simulink model "DHM"  (R2022a)
settings: Solver=FixedStepDiscrete  StartTime=0.0  StopTime=10.0  FixedStep=0.01  RelTol=1e-3
libraries: simulink x8, DoorHndReq x4, DoorHndDriver x2
settings Model: DataDictionary=DHM.sldd  Creator=liyun  LastModifiedBy=liyun
settings DataIOCC: SaveFormat=StructureWithTime
settings OptimizationCC: DefaultParameterBehavior=Inlined  EnhancedBackFolding=on  PassReuseOutputArgsAs=Individual arguments  ZeroExternalMemoryAtStartup=off  ZeroInternalMemoryAtStartup=off  OptimizeBlockOrder=speed  DifferentSizesBufferReuse=on  OptimizationCustomize=off  EfficientTunableParamExpr=on
settings DebuggingCC: ParameterTunabilityLossMsg=error
settings ModelReferenceCC: ModelReferenceNumInstancesAllowed=Single
settings SFSimCC: MATLABDynamicMemAlloc=off
settings RTWCC: Description=AUTOSAR  SystemTargetFile=autosar.tlc  GenCodeOnly=on  TemplateMakefile=ert_default_tmf
settings CodeAppCC: ForceParamTrailComments=on  IgnoreCustomStorageClasses=off  OperatorAnnotations=on  SimulinkDataObjDesc=on  SFDataObjDesc=on  InsertBlockDesc=on
settings STFCustomTargetCC: TargetLangStandard=C99 (ISO)  MultiwordLength=256  ParMdlRefBuildCompliant=on  CompOptLevelCompliant=on  IncludeMdlTerminateFcn=off  CombineOutputUpdateFcns=on  SuppressErrorStatus=on  ERTCustomFileBanners=on  SupportNonFinite=off  SupportComplex=off  SupportContinuousTime=off  SupportNonInlinedSFcns=off  RemoveResetFunc=on  MATLABClassNameForMDSCustomization=Simulink.SoftwareTarget.ERTCustomization  AutosarCompliant=on  GRTInterface=off  UseToolchainInfoCompliant=on  LookupTableObjectStructAxisOrder=2,1,3,4,...  LUTObjectStructOrderEvenSpacing=Size,Table,Breakpoints  SystemTargetFile=autosar.tlc
settings ERTTargetCC: TargetLangStandard=C99 (ISO)  ConcurrentExecutionCompliant=off  IncludeMdlTerminateFcn=off  SuppressErrorStatus=on  SupportNonFinite=off  SupportComplex=off  ModelStepFunctionPrototypeControlCompliant=off  CPPClassGenCompliant=off  AutosarCompliant=on  LookupTableObjectStructAxisOrder=2,1,3,4,...  LUTObjectStructOrderEvenSpacing=Size,Table,Breakpoints  InlinedParameterPlacement=NonHierarchical  ERTCustomFileTemplate=example_file_process.tlc

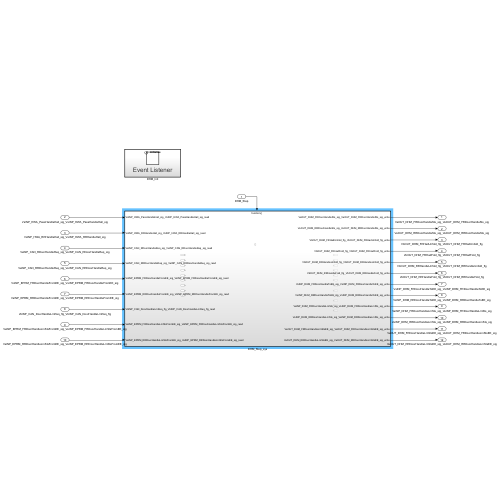
[thumbnail: Simulink's stored preview of the top-level diagram]
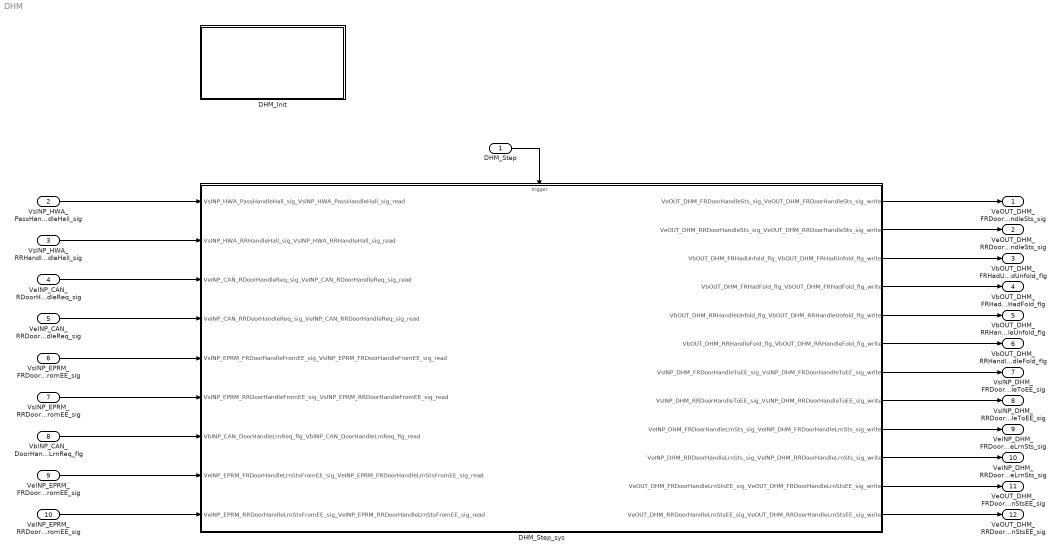
== system DHM ==
  DHM_Step : Inport  SampleTime=0.01  OutputFunctionCall=on
  VsINP_HWA_PassHandleHall_sig_VsINP_HWA_PassHandleHall_sig : Inport  Port=2  OutDataTypeStr=SInt16  PortDimensions=1
  VsINP_HWA_RRHandleHall_sig_VsINP_HWA_RRHandleHall_sig : Inport  Port=3  OutDataTypeStr=SInt16  PortDimensions=1
  VeINP_CAN_RDoorHandleReq_sig_VeINP_CAN_RDoorHandleReq_sig : Inport  Port=4  OutDataTypeStr=UInt8  PortDimensions=1
  VeINP_CAN_RRDoorHandleReq_sig_VeINP_CAN_RRDoorHandleReq_sig : Inport  Port=5  OutDataTypeStr=UInt8  PortDimensions=1
  VsINP_EPRM_FRDoorHandleFromEE_sig_VsINP_EPRM_FRDoorHandleFromEE_sig : Inport  Port=6  OutDataTypeStr=SInt16  PortDimensions=1
  VsINP_EPRM_RRDoorHandleFromEE_sig_VsINP_EPRM_RRDoorHandleFromEE_sig : Inport  Port=7  OutDataTypeStr=SInt16  PortDimensions=1
  VbINP_CAN_DoorHandleLrnReq_flg_VbINP_CAN_DoorHandleLrnReq_flg : Inport  Port=8  OutDataTypeStr=Boolean  PortDimensions=1
  VeINP_EPRM_FRDoorHandleLrnStsFromEE_sig_VeINP_EPRM_FRDoorHandleLrnStsFromEE_sig : Inport  Port=9  OutDataTypeStr=UInt8  PortDimensions=1
  VeINP_EPRM_RRDoorHandleLrnStsFromEE_sig_VeINP_EPRM_RRDoorHandleLrnStsFromEE_sig : Inport  Port=10  OutDataTypeStr=UInt8  PortDimensions=1
  DHM_Init : Subsystem
  DHM_Step_sys : Subsystem
  VeOUT_DHM_FRDoorHandleSts_sig_VeOUT_DHM_FRDoorHandleSts_sig : Outport  OutDataTypeStr=UInt8  PortDimensions=1
  VeOUT_DHM_RRDoorHandleSts_sig_VeOUT_DHM_RRDoorHandleSts_sig : Outport  Port=2  OutDataTypeStr=UInt8  PortDimensions=1
  VbOUT_DHM_FRHadUnfold_flg_VbOUT_DHM_FRHadUnfold_flg : Outport  Port=3  OutDataTypeStr=Boolean  PortDimensions=1
  VbOUT_DHM_FRHadFold_flg_VbOUT_DHM_FRHadFold_flg : Outport  Port=4  OutDataTypeStr=Boolean  PortDimensions=1
  VbOUT_DHM_RRHandleUnfold_flg_VbOUT_DHM_RRHandleUnfold_flg : Outport  Port=5  OutDataTypeStr=Boolean  PortDimensions=1
  VbOUT_DHM_RRHandleFold_flg_VbOUT_DHM_RRHandleFold_flg : Outport  Port=6  OutDataTypeStr=Boolean  PortDimensions=1
  VsINP_DHM_FRDoorHandleToEE_sig_VsINP_DHM_FRDoorHandleToEE_sig : Outport  Port=7  OutDataTypeStr=SInt16  PortDimensions=1
  VsINP_DHM_RRDoorHandleToEE_sig_VsINP_DHM_RRDoorHandleToEE_sig : Outport  Port=8  OutDataTypeStr=SInt16  PortDimensions=1
  VeINP_DHM_FRDoorHandleLrnSts_sig_VeINP_DHM_FRDoorHandleLrnSts_sig : Outport  Port=9  OutDataTypeStr=UInt8  PortDimensions=1
  VeINP_DHM_RRDoorHandleLrnSts_sig_VeINP_DHM_RRDoorHandleLrnSts_sig : Outport  Port=10  OutDataTypeStr=UInt8  PortDimensions=1
  VeOUT_DHM_FRDoorHandleLrnStsEE_sig_VeOUT_DHM_FRDoorHandleLrnStsEE_sig : Outport  Port=11  OutDataTypeStr=UInt8  PortDimensions=1
  VeOUT_DHM_RRDoorHandleLrnStsEE_sig_VeOUT_DHM_RRDoorHandleLrnStsEE_sig : Outport  Port=12  OutDataTypeStr=UInt8  PortDimensions=1
  wires:
  VsINP_HWA_PassHandleHall_sig_VsINP_HWA_PassHandleHall_sig/1 -> DHM_Step_sys/1(VsINP_HWA_PassHandleHall_sig_VsINP_HWA_PassHandleHall_sig_read)
  VsINP_HWA_RRHandleHall_sig_VsINP_HWA_RRHandleHall_sig/1 -> DHM_Step_sys/2(VsINP_HWA_RRHandleHall_sig_VsINP_HWA_RRHandleHall_sig_read)
  VeINP_CAN_RDoorHandleReq_sig_VeINP_CAN_RDoorHandleReq_sig/1 -> DHM_Step_sys/3(VeINP_CAN_RDoorHandleReq_sig_VeINP_CAN_RDoorHandleReq_sig_read)
  VeINP_CAN_RRDoorHandleReq_sig_VeINP_CAN_RRDoorHandleReq_sig/1 -> DHM_Step_sys/4(VeINP_CAN_RRDoorHandleReq_sig_VeINP_CAN_RRDoorHandleReq_sig_read)
  VsINP_EPRM_FRDoorHandleFromEE_sig_VsINP_EPRM_FRDoorHandleFromEE_sig/1 -> DHM_Step_sys/5(VsINP_EPRM_FRDoorHandleFromEE_sig_VsINP_EPRM_FRDoorHandleFromEE_sig_read)
  VsINP_EPRM_RRDoorHandleFromEE_sig_VsINP_EPRM_RRDoorHandleFromEE_sig/1 -> DHM_Step_sys/6(VsINP_EPRM_RRDoorHandleFromEE_sig_VsINP_EPRM_RRDoorHandleFromEE_sig_read)
  VbINP_CAN_DoorHandleLrnReq_flg_VbINP_CAN_DoorHandleLrnReq_flg/1 -> DHM_Step_sys/7(VbINP_CAN_DoorHandleLrnReq_flg_VbINP_CAN_DoorHandleLrnReq_flg_read)
  VeINP_EPRM_FRDoorHandleLrnStsFromEE_sig_VeINP_EPRM_FRDoorHandleLrnStsFromEE_sig/1 -> DHM_Step_sys/8(VeINP_EPRM_FRDoorHandleLrnStsFromEE_sig_VeINP_EPRM_FRDoorHandleLrnStsFromEE_sig_read)
  VeINP_EPRM_RRDoorHandleLrnStsFromEE_sig_VeINP_EPRM_RRDoorHandleLrnStsFromEE_sig/1 -> DHM_Step_sys/9(VeINP_EPRM_RRDoorHandleLrnStsFromEE_sig_VeINP_EPRM_RRDoorHandleLrnStsFromEE_sig_read)
  DHM_Step_sys/1(VeOUT_DHM_FRDoorHandleSts_sig_VeOUT_DHM_FRDoorHandleSts_sig_write) -> VeOUT_DHM_FRDoorHandleSts_sig_VeOUT_DHM_FRDoorHandleSts_sig/1
  DHM_Step_sys/2(VeOUT_DHM_RRDoorHandleSts_sig_VeOUT_DHM_RRDoorHandleSts_sig_write) -> VeOUT_DHM_RRDoorHandleSts_sig_VeOUT_DHM_RRDoorHandleSts_sig/1
  DHM_Step_sys/3(VbOUT_DHM_FRHadUnfold_flg_VbOUT_DHM_FRHadUnfold_flg_write) -> VbOUT_DHM_FRHadUnfold_flg_VbOUT_DHM_FRHadUnfold_flg/1
  DHM_Step_sys/4(VbOUT_DHM_FRHadFold_flg_VbOUT_DHM_FRHadFold_flg_write) -> VbOUT_DHM_FRHadFold_flg_VbOUT_DHM_FRHadFold_flg/1
  DHM_Step_sys/5(VbOUT_DHM_RRHandleUnfold_flg_VbOUT_DHM_RRHandleUnfold_flg_write) -> VbOUT_DHM_RRHandleUnfold_flg_VbOUT_DHM_RRHandleUnfold_flg/1
  DHM_Step_sys/6(VbOUT_DHM_RRHandleFold_flg_VbOUT_DHM_RRHandleFold_flg_write) -> VbOUT_DHM_RRHandleFold_flg_VbOUT_DHM_RRHandleFold_flg/1
  DHM_Step_sys/7(VsINP_DHM_FRDoorHandleToEE_sig_VsINP_DHM_FRDoorHandleToEE_sig_write) -> VsINP_DHM_FRDoorHandleToEE_sig_VsINP_DHM_FRDoorHandleToEE_sig/1
  DHM_Step_sys/8(VsINP_DHM_RRDoorHandleToEE_sig_VsINP_DHM_RRDoorHandleToEE_sig_write) -> VsINP_DHM_RRDoorHandleToEE_sig_VsINP_DHM_RRDoorHandleToEE_sig/1
  DHM_Step_sys/9(VeINP_DHM_FRDoorHandleLrnSts_sig_VeINP_DHM_FRDoorHandleLrnSts_sig_write) -> VeINP_DHM_FRDoorHandleLrnSts_sig_VeINP_DHM_FRDoorHandleLrnSts_sig/1
  DHM_Step_sys/10(VeINP_DHM_RRDoorHandleLrnSts_sig_VeINP_DHM_RRDoorHandleLrnSts_sig_write) -> VeINP_DHM_RRDoorHandleLrnSts_sig_VeINP_DHM_RRDoorHandleLrnSts_sig/1
  DHM_Step_sys/11(VeOUT_DHM_FRDoorHandleLrnStsEE_sig_VeOUT_DHM_FRDoorHandleLrnStsEE_sig_write) -> VeOUT_DHM_FRDoorHandleLrnStsEE_sig_VeOUT_DHM_FRDoorHandleLrnStsEE_sig/1
  DHM_Step_sys/12(VeOUT_DHM_RRDoorHandleLrnStsEE_sig_VeOUT_DHM_RRDoorHandleLrnStsEE_sig_write) -> VeOUT_DHM_RRDoorHandleLrnStsEE_sig_VeOUT_DHM_RRDoorHandleLrnStsEE_sig/1
  DHM_Step/1 -> DHM_Step_sys/Trigger

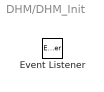
== system DHM/DHM_Init ==
  Event Listener : EventListener  EventName=reset

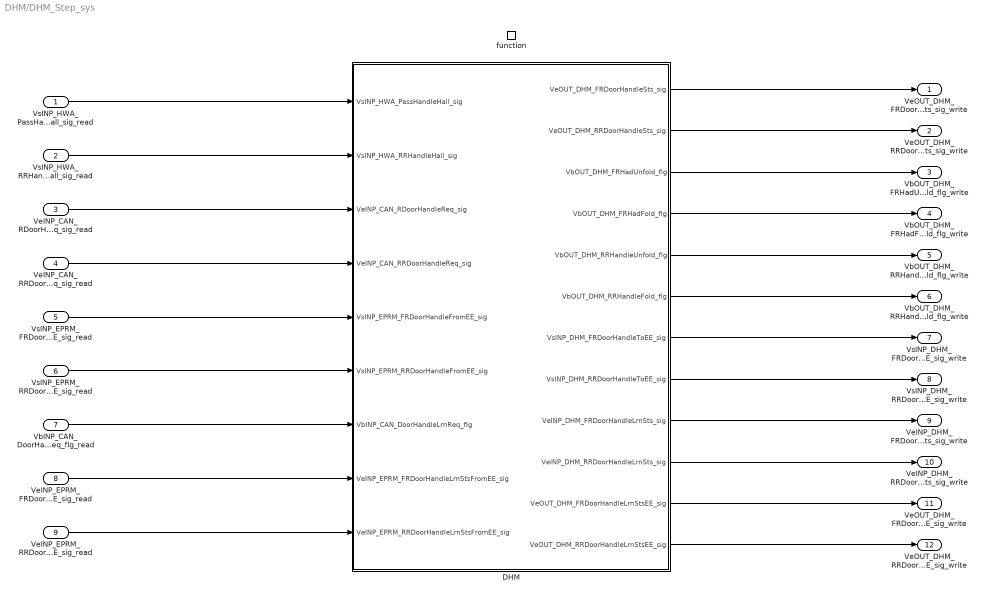
== system DHM/DHM_Step_sys ==
  VsINP_HWA_PassHandleHall_sig_VsINP_HWA_PassHandleHall_sig_read : Inport
  VsINP_HWA_RRHandleHall_sig_VsINP_HWA_RRHandleHall_sig_read : Inport  Port=2
  VeINP_CAN_RDoorHandleReq_sig_VeINP_CAN_RDoorHandleReq_sig_read : Inport  Port=3
  VeINP_CAN_RRDoorHandleReq_sig_VeINP_CAN_RRDoorHandleReq_sig_read : Inport  Port=4
  VsINP_EPRM_FRDoorHandleFromEE_sig_VsINP_EPRM_FRDoorHandleFromEE_sig_read : Inport  Port=5
  VsINP_EPRM_RRDoorHandleFromEE_sig_VsINP_EPRM_RRDoorHandleFromEE_sig_read : Inport  Port=6
  VbINP_CAN_DoorHandleLrnReq_flg_VbINP_CAN_DoorHandleLrnReq_flg_read : Inport  Port=7
  VeINP_EPRM_FRDoorHandleLrnStsFromEE_sig_VeINP_EPRM_FRDoorHandleLrnStsFromEE_sig_read : Inport  Port=8
  VeINP_EPRM_RRDoorHandleLrnStsFromEE_sig_VeINP_EPRM_RRDoorHandleLrnStsFromEE_sig_read : Inport  Port=9
  function : TriggerPort  TriggerType=function-call  VariantControl=(inherit)  SampleTimeType=periodic  SampleTime=-1
  DHM : Subsystem
  VeOUT_DHM_FRDoorHandleSts_sig_VeOUT_DHM_FRDoorHandleSts_sig_write : Outport
      settings: EnsureOutportIsVirtual=on
  VeOUT_DHM_RRDoorHandleSts_sig_VeOUT_DHM_RRDoorHandleSts_sig_write : Outport  Port=2
      settings: EnsureOutportIsVirtual=on
  VbOUT_DHM_FRHadUnfold_flg_VbOUT_DHM_FRHadUnfold_flg_write : Outport  Port=3
      settings: EnsureOutportIsVirtual=on
  VbOUT_DHM_FRHadFold_flg_VbOUT_DHM_FRHadFold_flg_write : Outport  Port=4
      settings: EnsureOutportIsVirtual=on
  VbOUT_DHM_RRHandleUnfold_flg_VbOUT_DHM_RRHandleUnfold_flg_write : Outport  Port=5
      settings: EnsureOutportIsVirtual=on
  VbOUT_DHM_RRHandleFold_flg_VbOUT_DHM_RRHandleFold_flg_write : Outport  Port=6
      settings: EnsureOutportIsVirtual=on
  VsINP_DHM_FRDoorHandleToEE_sig_VsINP_DHM_FRDoorHandleToEE_sig_write : Outport  Port=7
      settings: EnsureOutportIsVirtual=on
  VsINP_DHM_RRDoorHandleToEE_sig_VsINP_DHM_RRDoorHandleToEE_sig_write : Outport  Port=8
      settings: EnsureOutportIsVirtual=on
  VeINP_DHM_FRDoorHandleLrnSts_sig_VeINP_DHM_FRDoorHandleLrnSts_sig_write : Outport  Port=9
      settings: EnsureOutportIsVirtual=on
  VeINP_DHM_RRDoorHandleLrnSts_sig_VeINP_DHM_RRDoorHandleLrnSts_sig_write : Outport  Port=10
      settings: EnsureOutportIsVirtual=on
  VeOUT_DHM_FRDoorHandleLrnStsEE_sig_VeOUT_DHM_FRDoorHandleLrnStsEE_sig_write : Outport  Port=11
      settings: EnsureOutportIsVirtual=on
  VeOUT_DHM_RRDoorHandleLrnStsEE_sig_VeOUT_DHM_RRDoorHandleLrnStsEE_sig_write : Outport  Port=12
      settings: EnsureOutportIsVirtual=on
  wires:
  VsINP_HWA_PassHandleHall_sig_VsINP_HWA_PassHandleHall_sig_read/1 -> DHM/1(VsINP_HWA_PassHandleHall_sig)
  VsINP_HWA_RRHandleHall_sig_VsINP_HWA_RRHandleHall_sig_read/1 -> DHM/2(VsINP_HWA_RRHandleHall_sig)
  VeINP_CAN_RDoorHandleReq_sig_VeINP_CAN_RDoorHandleReq_sig_read/1 -> DHM/3(VeINP_CAN_RDoorHandleReq_sig)
  VeINP_CAN_RRDoorHandleReq_sig_VeINP_CAN_RRDoorHandleReq_sig_read/1 -> DHM/4(VeINP_CAN_RRDoorHandleReq_sig)
  VsINP_EPRM_FRDoorHandleFromEE_sig_VsINP_EPRM_FRDoorHandleFromEE_sig_read/1 -> DHM/5(VsINP_EPRM_FRDoorHandleFromEE_sig)
  VsINP_EPRM_RRDoorHandleFromEE_sig_VsINP_EPRM_RRDoorHandleFromEE_sig_read/1 -> DHM/6(VsINP_EPRM_RRDoorHandleFromEE_sig)
  VbINP_CAN_DoorHandleLrnReq_flg_VbINP_CAN_DoorHandleLrnReq_flg_read/1 -> DHM/7(VbINP_CAN_DoorHandleLrnReq_flg)
  VeINP_EPRM_FRDoorHandleLrnStsFromEE_sig_VeINP_EPRM_FRDoorHandleLrnStsFromEE_sig_read/1 -> DHM/8(VeINP_EPRM_FRDoorHandleLrnStsFromEE_sig)
  VeINP_EPRM_RRDoorHandleLrnStsFromEE_sig_VeINP_EPRM_RRDoorHandleLrnStsFromEE_sig_read/1 -> DHM/9(VeINP_EPRM_RRDoorHandleLrnStsFromEE_sig)
  DHM/2(VeOUT_DHM_RRDoorHandleSts_sig) -> VeOUT_DHM_RRDoorHandleSts_sig_VeOUT_DHM_RRDoorHandleSts_sig_write/1
  DHM/3(VbOUT_DHM_FRHadUnfold_flg) -> VbOUT_DHM_FRHadUnfold_flg_VbOUT_DHM_FRHadUnfold_flg_write/1
  DHM/1(VeOUT_DHM_FRDoorHandleSts_sig) -> VeOUT_DHM_FRDoorHandleSts_sig_VeOUT_DHM_FRDoorHandleSts_sig_write/1
  DHM/4(VbOUT_DHM_FRHadFold_flg) -> VbOUT_DHM_FRHadFold_flg_VbOUT_DHM_FRHadFold_flg_write/1
  DHM/5(VbOUT_DHM_RRHandleUnfold_flg) -> VbOUT_DHM_RRHandleUnfold_flg_VbOUT_DHM_RRHandleUnfold_flg_write/1
  DHM/6(VbOUT_DHM_RRHandleFold_flg) -> VbOUT_DHM_RRHandleFold_flg_VbOUT_DHM_RRHandleFold_flg_write/1
  DHM/7(VsINP_DHM_FRDoorHandleToEE_sig) -> VsINP_DHM_FRDoorHandleToEE_sig_VsINP_DHM_FRDoorHandleToEE_sig_write/1
  DHM/8(VsINP_DHM_RRDoorHandleToEE_sig) -> VsINP_DHM_RRDoorHandleToEE_sig_VsINP_DHM_RRDoorHandleToEE_sig_write/1
  DHM/9(VeINP_DHM_FRDoorHandleLrnSts_sig) -> VeINP_DHM_FRDoorHandleLrnSts_sig_VeINP_DHM_FRDoorHandleLrnSts_sig_write/1
  DHM/10(VeINP_DHM_RRDoorHandleLrnSts_sig) -> VeINP_DHM_RRDoorHandleLrnSts_sig_VeINP_DHM_RRDoorHandleLrnSts_sig_write/1
  DHM/11(VeOUT_DHM_FRDoorHandleLrnStsEE_sig) -> VeOUT_DHM_FRDoorHandleLrnStsEE_sig_VeOUT_DHM_FRDoorHandleLrnStsEE_sig_write/1
  DHM/12(VeOUT_DHM_RRDoorHandleLrnStsEE_sig) -> VeOUT_DHM_RRDoorHandleLrnStsEE_sig_VeOUT_DHM_RRDoorHandleLrnStsEE_sig_write/1

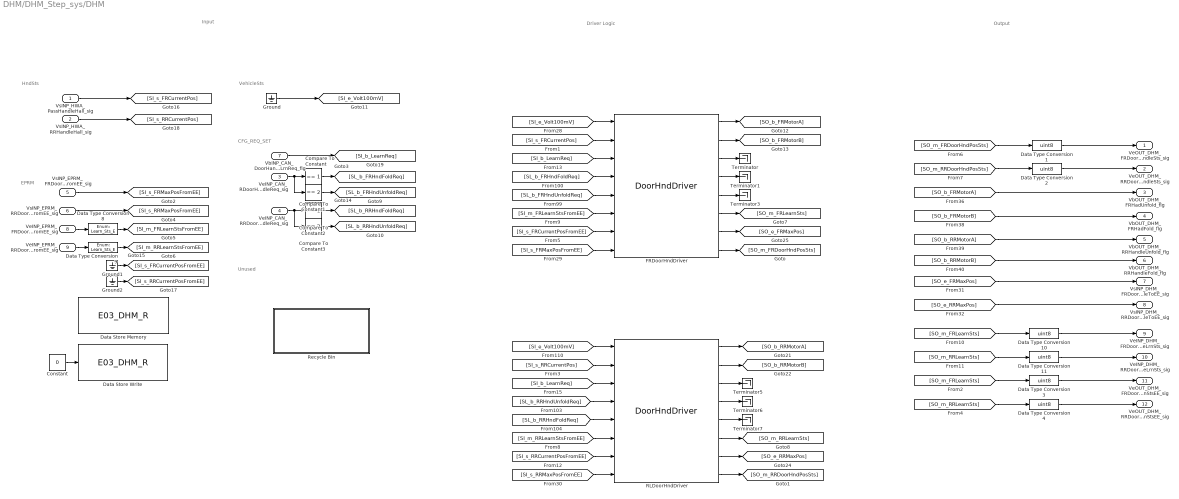
== system DHM/DHM_Step_sys/DHM ==
  note: HndSts
  note: Output
  note: Driver Logic
  note: Input
  note: VehicleSts
  note: Unused
  note: CFG_REQ_SET
  note: EPRM
  VsINP_HWA_PassHandleHall_sig : Inport
  VsINP_HWA_RRHandleHall_sig : Inport  Port=2
  VeINP_CAN_RDoorHandleReq_sig : Inport  Port=3
  VeINP_CAN_RRDoorHandleReq_sig : Inport  Port=4
  VsINP_EPRM_FRDoorHandleFromEE_sig : Inport  Port=5
  VsINP_EPRM_RRDoorHandleFromEE_sig : Inport  Port=6
  VbINP_CAN_DoorHandleLrnReq_flg : Inport  Port=7
  VeINP_EPRM_FRDoorHandleLrnStsFromEE_sig : Inport  Port=8
  VeINP_EPRM_RRDoorHandleLrnStsFromEE_sig : Inport  Port=9
  Compare To Constant : simulink/Logic and Bit Operations/Compare To Constant  relop===  const=1  OutDataTypeStr=boolean
  Compare To Constant1 : simulink/Logic and Bit Operations/Compare To Constant  relop===  const=2  OutDataTypeStr=boolean
  Compare To Constant2 : simulink/Logic and Bit Operations/Compare To Constant  relop===  const=1  OutDataTypeStr=boolean
  Compare To Constant3 : simulink/Logic and Bit Operations/Compare To Constant  relop===  const=2  OutDataTypeStr=boolean
  Constant : Constant  Value=0  OutDataTypeStr=uint8
  Data Store Memory : DataStoreMemory  DataStoreName=E03_DHM_R  WriteAfterWriteMsg=warning  ShowAdditionalParam=off  OutDataTypeStr=uint8
  Data Store Write : DataStoreWrite  DataStoreName=E03_DHM_R  IndexOptions=Index vector (dialog)  Indices=1  OutputSizes=1
  Data Type Conversion{1..4,10..11} (6 alike) : DataTypeConversion  OutDataTypeStr=uint8  SaturateOnIntegerOverflow=off  RndMeth=Floor
  Data Type Conversion8 : DataTypeConversion  OutDataTypeStr=Enum: Learn_Sts_E  SaturateOnIntegerOverflow=off  RndMeth=Floor
  Data Type Conversion9 : DataTypeConversion  OutDataTypeStr=Enum: Learn_Sts_E  SaturateOnIntegerOverflow=off  RndMeth=Floor
  FRDoorHndDriver : DoorHndDriver/DoorHndDriver  SystemSampleTime=-1  VariantActivationTime=update diagram  Latency=0  AutoFrameSizeCalculation=off
  Ground : Ground
  Ground1 : Ground
  Ground2 : Ground
  RLDoorHndDriver : DoorHndDriver/DoorHndDriver  SystemSampleTime=-1  VariantActivationTime=update diagram  Latency=0  AutoFrameSizeCalculation=off
  Recycle Bin : Subsystem
  Terminator{,1,3,5..7} (6 alike) : Terminator
  VeOUT_DHM_FRDoorHandleSts_sig : Outport
  VeOUT_DHM_RRDoorHandleSts_sig : Outport  Port=2
  VbOUT_DHM_FRHadUnfold_flg : Outport  Port=3
  VbOUT_DHM_FRHadFold_flg : Outport  Port=4
  VbOUT_DHM_RRHandleUnfold_flg : Outport  Port=5
  VbOUT_DHM_RRHandleFold_flg : Outport  Port=6
  VsINP_DHM_FRDoorHandleToEE_sig : Outport  Port=7
  VsINP_DHM_RRDoorHandleToEE_sig : Outport  Port=8
  VeINP_DHM_FRDoorHandleLrnSts_sig : Outport  Port=9
  VeINP_DHM_RRDoorHandleLrnSts_sig : Outport  Port=10
  VeOUT_DHM_FRDoorHandleLrnStsEE_sig : Outport  Port=11
  VeOUT_DHM_RRDoorHandleLrnStsEE_sig : Outport  Port=12
  wires:
  [SI_e_Volt100mV] -> FRDoorHndDriver/1
  [SI_e_Volt100mV] -> RLDoorHndDriver/1
  Ground/1 -> [SI_e_Volt100mV]
  Constant/1 -> Data Store Write/1
  VsINP_HWA_PassHandleHall_sig/1 -> [SI_s_FRCurrentPos]
  VsINP_HWA_RRHandleHall_sig/1 -> [SI_s_RRCurrentPos]
  [SI_s_FRCurrentPos] -> FRDoorHndDriver/2
  [SI_s_RRCurrentPos] -> RLDoorHndDriver/2
  VbINP_CAN_DoorHandleLrnReq_flg/1 -> [SI_b_LearnReq]
  [SI_b_LearnReq] -> FRDoorHndDriver/3
  [SI_b_LearnReq] -> RLDoorHndDriver/3
  VsINP_EPRM_FRDoorHandleFromEE_sig/1 -> [SI_s_FRMaxPosFromEE]
  VsINP_EPRM_RRDoorHandleFromEE_sig/1 -> [SI_s_RRMaxPosFromEE]
  [SO_e_RRMaxPos] -> VsINP_DHM_RRDoorHandleToEE_sig/1
  [SO_e_FRMaxPos] -> VsINP_DHM_FRDoorHandleToEE_sig/1
  [SO_b_FRMotorA] -> VbOUT_DHM_FRHadUnfold_flg/1
  [SO_b_FRMotorB] -> VbOUT_DHM_FRHadFold_flg/1
  [SO_b_RRMotorA] -> VbOUT_DHM_RRHandleUnfold_flg/1
  [SO_b_RRMotorB] -> VbOUT_DHM_RRHandleFold_flg/1
  FRDoorHndDriver/1 -> [SO_b_FRMotorA]
  FRDoorHndDriver/2 -> [SO_b_FRMotorB]
  [SI_m_FRLearnStsFromEE] -> FRDoorHndDriver/6
  [SL_b_FRHndUnfoldReq] -> FRDoorHndDriver/5
  [SL_b_FRHndFoldReq] -> FRDoorHndDriver/4
  [SI_m_RRLearnStsFromEE] -> RLDoorHndDriver/6
  [SL_b_RRHndFoldReq] -> RLDoorHndDriver/5
  [SL_b_RRHndUnfoldReq] -> RLDoorHndDriver/4
  RLDoorHndDriver/1 -> [SO_b_RRMotorA]
  RLDoorHndDriver/2 -> [SO_b_RRMotorB]
  [SO_m_FRDoorHndPosSts] -> Data Type Conversion1/1
  Data Type Conversion1/1 -> VeOUT_DHM_FRDoorHandleSts_sig/1
  Data Type Conversion2/1 -> VeOUT_DHM_RRDoorHandleSts_sig/1
  [SO_m_RRDoorHndPosSts] -> Data Type Conversion2/1
  VeINP_EPRM_FRDoorHandleLrnStsFromEE_sig/1 -> Data Type Conversion8/1
  Data Type Conversion8/1 -> [SI_m_FRLearnStsFromEE]
  VeINP_EPRM_RRDoorHandleLrnStsFromEE_sig/1 -> Data Type Conversion9/1
  Data Type Conversion9/1 -> [SI_m_RRLearnStsFromEE]
  [SO_m_FRLearnSts] -> Data Type Conversion10/1
  Data Type Conversion10/1 -> VeINP_DHM_FRDoorHandleLrnSts_sig/1
  [SO_m_RRLearnSts] -> Data Type Conversion11/1
  Data Type Conversion11/1 -> VeINP_DHM_RRDoorHandleLrnSts_sig/1
  VeINP_CAN_RDoorHandleReq_sig/1 -> Compare To Constant1/1, Compare To Constant/1
  Compare To Constant/1 -> [SL_b_FRHndFoldReq]
  Compare To Constant1/1 -> [SL_b_FRHndUnfoldReq]
  Compare To Constant3/1 -> [SL_b_RRHndUnfoldReq]
  Compare To Constant2/1 -> [SL_b_RRHndFoldReq]
  VeINP_CAN_RRDoorHandleReq_sig/1 -> Compare To Constant3/1, Compare To Constant2/1
  Data Type Conversion3/1 -> VeOUT_DHM_FRDoorHandleLrnStsEE_sig/1
  [SO_m_RRLearnSts] -> Data Type Conversion4/1
  Data Type Conversion4/1 -> VeOUT_DHM_RRDoorHandleLrnStsEE_sig/1
  [SO_m_FRLearnSts] -> Data Type Conversion3/1
  RLDoorHndDriver/3 -> Terminator5/1
  RLDoorHndDriver/4 -> Terminator6/1
  FRDoorHndDriver/3 -> Terminator/1
  FRDoorHndDriver/4 -> Terminator1/1
  FRDoorHndDriver/7 -> [SO_e_FRMaxPos]
  FRDoorHndDriver/6 -> [SO_m_FRLearnSts]
  FRDoorHndDriver/8 -> [SO_m_FRDoorHndPosSts]
  FRDoorHndDriver/5 -> Terminator3/1
  [SI_s_FRMaxPosFromEE] -> FRDoorHndDriver/8
  [SI_s_FRCurrentPosFromEE] -> FRDoorHndDriver/7
  RLDoorHndDriver/7 -> [SO_e_RRMaxPos]
  RLDoorHndDriver/6 -> [SO_m_RRLearnSts]
  RLDoorHndDriver/8 -> [SO_m_RRDoorHndPosSts]
  RLDoorHndDriver/5 -> Terminator7/1
  [SI_s_RRCurrentPosFromEE] -> RLDoorHndDriver/7
  [SI_s_RRMaxPosFromEE] -> RLDoorHndDriver/8
  Ground2/1 -> [SI_s_RRCurrentPosFromEE]
  Ground1/1 -> [SI_s_FRCurrentPosFromEE]

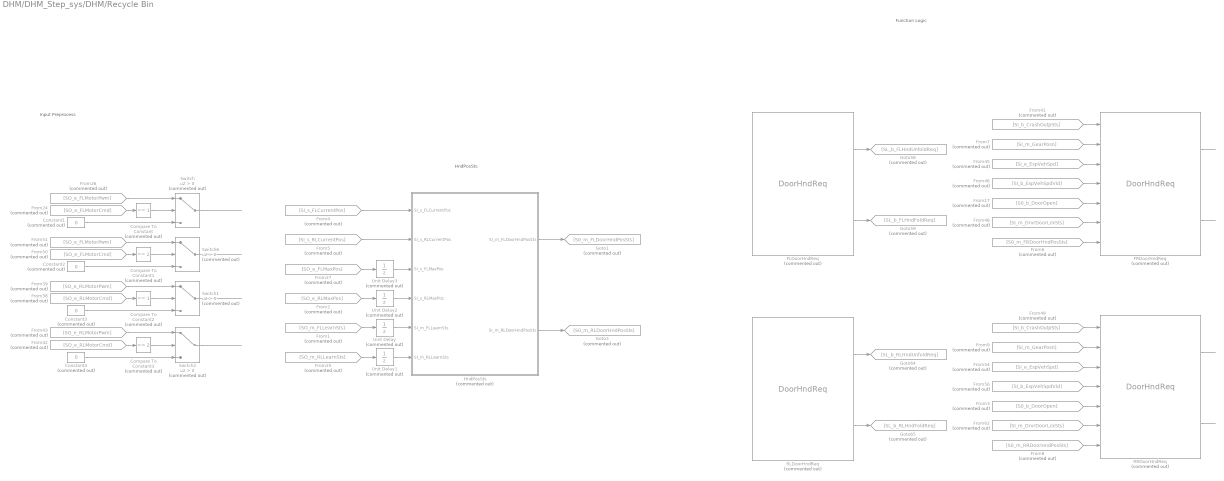
== system DHM/DHM_Step_sys/DHM/Recycle Bin ==
  note: Input Preprocess
  note: HndPosSts
  note: Function Logic
  Compare To Constant : simulink/Logic and Bit Operations/Compare To Constant  Commented=on  relop===  const=1  OutDataTypeStr=boolean
  Compare To Constant1 : simulink/Logic and Bit Operations/Compare To Constant  Commented=on  relop===  const=2  OutDataTypeStr=boolean
  Compare To Constant2 : simulink/Logic and Bit Operations/Compare To Constant  Commented=on  relop===  const=1  OutDataTypeStr=boolean
  Compare To Constant3 : simulink/Logic and Bit Operations/Compare To Constant  Commented=on  relop===  const=2  OutDataTypeStr=boolean
  Constant{1..4} (4 alike) : Constant  Commented=on  Value=0
  FLDoorHndReq : DoorHndReq/DoorHndReq  Commented=on  SystemSampleTime=-1  VariantActivationTime=update diagram  Latency=0  AutoFrameSizeCalculation=off
  FRDoorHndReq : DoorHndReq/DoorHndReq  Commented=on  SystemSampleTime=-1  VariantActivationTime=update diagram  Latency=0  AutoFrameSizeCalculation=off
  From1 : From  Commented=on  GotoTag=SO_m_FLLearnSts
  From17 : From  Commented=on  GotoTag=S0_b_DoorOpen
  From2 : From  Commented=on  GotoTag=SO_e_RLMaxPos
  From24 : From  Commented=on  GotoTag=SO_e_FLMotorCmd
  From25 : From  Commented=on  GotoTag=SO_m_RLLearnSts
  From26 : From  Commented=on  GotoTag=SO_e_FLMotorPwm
  From27 : From  Commented=on  GotoTag=SO_e_FLMaxPos
  From3 : From  Commented=on  GotoTag=S0_b_DoorOpen
  From38 : From  Commented=on  GotoTag=SO_e_RLMotorCmd
  From39 : From  Commented=on  GotoTag=SO_e_RLMotorPwm
  From4 : From  Commented=on  GotoTag=SI_s_FLCurrentPos
  From41 : From  Commented=on  GotoTag=SI_b_CrashOutpSts
  From42 : From  Commented=on  GotoTag=SO_e_RLMotorCmd
  From43 : From  Commented=on  GotoTag=SO_e_RLMotorPwm
  From45 : From  Commented=on  GotoTag=SI_e_EspVehSpd
  From46 : From  Commented=on  GotoTag=SI_b_EspVehSpdVld
  From48 : From  Commented=on  GotoTag=SI_m_DrvrDoorLckSts
  From49 : From  Commented=on  GotoTag=SI_b_CrashOutpSts
  From5 : From  Commented=on  GotoTag=SI_s_RLCurrentPos
  From50 : From  Commented=on  GotoTag=SO_e_FLMotorCmd
  From51 : From  Commented=on  GotoTag=SO_e_FLMotorPwm
  From54 : From  Commented=on  GotoTag=SI_e_EspVehSpd
  From56 : From  Commented=on  GotoTag=SI_b_EspVehSpdVld
  From6 : From  Commented=on  GotoTag=S0_m_FRDoorHndPosSts
  From62 : From  Commented=on  GotoTag=SI_m_DrvrDoorLckSts
  From7 : From  Commented=on  GotoTag=SI_m_GearPosn
  From8 : From  Commented=on  GotoTag=S0_m_RRDoorHndPosSts
  From9 : From  Commented=on  GotoTag=SI_m_GearPosn
  Goto1 : Goto  Commented=on  GotoTag=S0_m_FLDoorHndPosSts
  Goto3 : Goto  Commented=on  GotoTag=S0_m_RLDoorHndPosSts
  Goto58 : Goto  Commented=on  GotoTag=SL_b_FLHndUnfoldReq
  Goto59 : Goto  Commented=on  GotoTag=SL_b_FLHndFoldReq
  Goto64 : Goto  Commented=on  GotoTag=SL_b_RLHndUnfoldReq
  Goto65 : Goto  Commented=on  GotoTag=SL_b_RLHndFoldReq
  HndPosSts : Stateflow chart  Commented=on  TreatAsAtomicUnit=on
  RLDoorHndReq : DoorHndReq/DoorHndReq  Commented=on  SystemSampleTime=-1  VariantActivationTime=update diagram  Latency=0  AutoFrameSizeCalculation=off
  RRDoorHndReq : DoorHndReq/DoorHndReq  Commented=on  SystemSampleTime=-1  VariantActivationTime=update diagram  Latency=0  AutoFrameSizeCalculation=off
  Switch{,1..2,6} (4 alike) : Switch  Commented=on  Criteria=u2 > Threshold  SaturateOnIntegerOverflow=off  InputSameDT=off
  Unit Delay{,1..3} (4 alike) : UnitDelay  Commented=on  SampleTime=-1  HasFrameUpgradeWarning=on
  wires:
  Switch/1 -> ?
  Switch1/1 -> ?
  Switch2/1 -> ?
  Switch6/1 -> ?
  From43/1 -> Switch2/1
  Constant1/1 -> Switch/3
  Constant4/1 -> Switch2/3
  Constant3/1 -> Switch1/3
  From39/1 -> Switch1/1
  From50/1 -> Compare To Constant1/1
  From51/1 -> Switch6/1
  From26/1 -> Switch/1
  Constant2/1 -> Switch6/3
  From38/1 -> Compare To Constant2/1
  Compare To Constant3/1 -> Switch2/2
  From42/1 -> Compare To Constant3/1
  Compare To Constant/1 -> Switch/2
  Compare To Constant2/1 -> Switch1/2
  Compare To Constant1/1 -> Switch6/2
  From24/1 -> Compare To Constant/1
  From25/1 -> Unit Delay1/1
  Unit Delay2/1 -> HndPosSts/4(SI_s_RLMaxPos)
  Unit Delay3/1 -> HndPosSts/3(SI_s_FLMaxPos)
  HndPosSts/2(SI_m_RLDoorHndPosSts) -> Goto3/1
  From4/1 -> HndPosSts/1(SI_s_FLCurrentPos)
  From27/1 -> Unit Delay3/1
  From2/1 -> Unit Delay2/1
  Unit Delay/1 -> HndPosSts/5(SI_m_FLLearnSts)
  Unit Delay1/1 -> HndPosSts/6(SI_m_RLLearnSts)
  HndPosSts/1(SI_m_FLDoorHndPosSts) -> Goto1/1
  From1/1 -> Unit Delay/1
  From5/1 -> HndPosSts/2(SI_s_RLCurrentPos)
  ? -> FLDoorHndReq/5
  From56/1 -> RRDoorHndReq/4
  ? -> FLDoorHndReq/3
  From41/1 -> FRDoorHndReq/1
  RRDoorHndReq/1 -> ?
  From7/1 -> FRDoorHndReq/2
  FRDoorHndReq/1 -> ?
  FRDoorHndReq/2 -> ?
  From45/1 -> FRDoorHndReq/3
  From9/1 -> RRDoorHndReq/2
  FLDoorHndReq/1 -> Goto58/1
  ? -> RLDoorHndReq/4
  RLDoorHndReq/1 -> Goto64/1
  From49/1 -> RRDoorHndReq/1
  ? -> FLDoorHndReq/2
  ? -> RLDoorHndReq/2
  FLDoorHndReq/2 -> Goto59/1
  RLDoorHndReq/2 -> Goto65/1
  From6/1 -> FRDoorHndReq/7
  From3/1 -> RRDoorHndReq/5
  ? -> RLDoorHndReq/5
  ? -> RLDoorHndReq/7
  RRDoorHndReq/2 -> ?
  ? -> FLDoorHndReq/6
  ? -> RLDoorHndReq/3
  ? -> FLDoorHndReq/7
  ? -> FLDoorHndReq/1
  ? -> RLDoorHndReq/6
  ? -> FLDoorHndReq/4
  From46/1 -> FRDoorHndReq/4
  From17/1 -> FRDoorHndReq/5
  From62/1 -> RRDoorHndReq/6
  ? -> RLDoorHndReq/1
  From8/1 -> RRDoorHndReq/7
  From54/1 -> RRDoorHndReq/3
  From48/1 -> FRDoorHndReq/6

== stateflow chart DHM/DHM_Step_sys/DHM/Recycle Bin/HndPosSts ==
  state GetSoftPos [parallel]
    settings: executionOrder=1
    (default) -> (junction 102)
    GetSoftPos -> (junction 102)
    (junction 102) -> (junction 103) [order 1] : [SI_m_FLLearnSts == Learn_Success]
    (junction 103) -> (junction 106) : {SL_s_FLMaxSoftPos = SI_s_FLMaxPos*95/100;
        | SL_s_FLMinSoftPos = SI_s_FLMaxPos*5/100;}
    (junction 102) -> (junction 106) [order 2]
    (junction 106) -> (junction 111)
    (junction 111) -> (junction 115) [order 1] : [SI_m_RLLearnSts == Learn_Success]
    (junction 115) -> (junction 117) : {SL_s_RLMaxSoftPos = SI_s_RLMaxPos*95/100;
        | SL_s_RLMinSoftPos = SI_s_RLMaxPos*5/100;}
    (junction 111) -> (junction 117) [order 2]
    (junction 117) -> (junction 120)
  state HndPosSts [parallel]
    settings: executionOrder=2
    (default) -> (junction 149)
    HndPosSts -> (junction 149)
    (junction 149) -> (junction 150) : {SI_m_FLDoorHndPosSts = GetPosSts(SI_s_FLCurrentPos, SL_s_FLMinSoftPos, SL_s_FLMaxSoftPos);}
    (junction 150) -> (junction 235)
    (junction 235) -> (junction 151) : {SI_m_RLDoorHndPosSts = GetPosSts(SI_s_RLCurrentPos, SL_s_RLMinSoftPos, SL_s_RLMaxSoftPos);}
    (junction 151) -> (junction 153)
  state y = GetPosSts(CurrentPos, MinSoftPos, MaxSoftPos) [function]
    (default) -> (junction 212)
    (junction 212) -> (junction 213) [order 1] : [CurrentPos <= MinSoftPos]
    (junction 212) -> (junction 229) [order 2]
    (junction 213) -> (junction 221) : {y = Hnd_Unfold;}
    (junction 229) -> (junction 219) [order 1] : [CurrentPos >=  MaxSoftPos]
    (junction 229) -> (junction 215) [order 2] : {y = Hnd_Unknown;}
    (junction 219) -> (junction 226) : {y = Hnd_Fold;}
    (junction 226) -> (junction 215)
    (junction 221) -> (junction 226)
    (junction 215) -> (junction 232)
  data: CurrentPos function_input double; y function_output double; MinSoftPos function_input double; MaxSoftPos function_input double; SI_m_FLDoorHndPosSts output Enum: HndPos_Sts_E; SI_m_RLDoorHndPosSts output Enum: HndPos_Sts_E; SI_s_FLCurrentPos input int16; SI_s_RLCurrentPos input int16; SI_s_FLMaxPos input int16; SI_s_RLMaxPos input int16; SI_m_FLLearnSts input Enum: Learn_Sts_E; SI_m_RLLearnSts input Enum: Learn_Sts_E; SL_s_FLMaxSoftPos local int16; SL_s_FLMinSoftPos local int16; SL_s_RLMaxSoftPos local int16; SL_s_RLMinSoftPos local int16
